simulink model "Kalman_builtin"  (R2024a)
settings: Solver=VariableStepAuto  StartTime=0.0  StopTime=10.0  RelTol=1e-3
undefined symbols (not defined in the file or in its folder): pInitialization
libraries: ctrlSharedLib x40, simulink x2
settings Model: Creator=DELL  LastModifiedBy=DELL

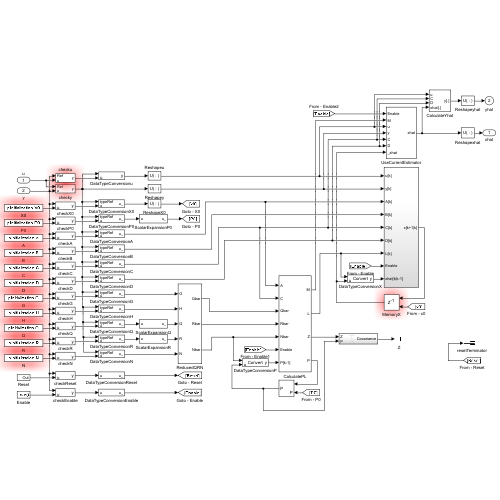
[thumbnail: Simulink's stored preview of the top-level diagram]
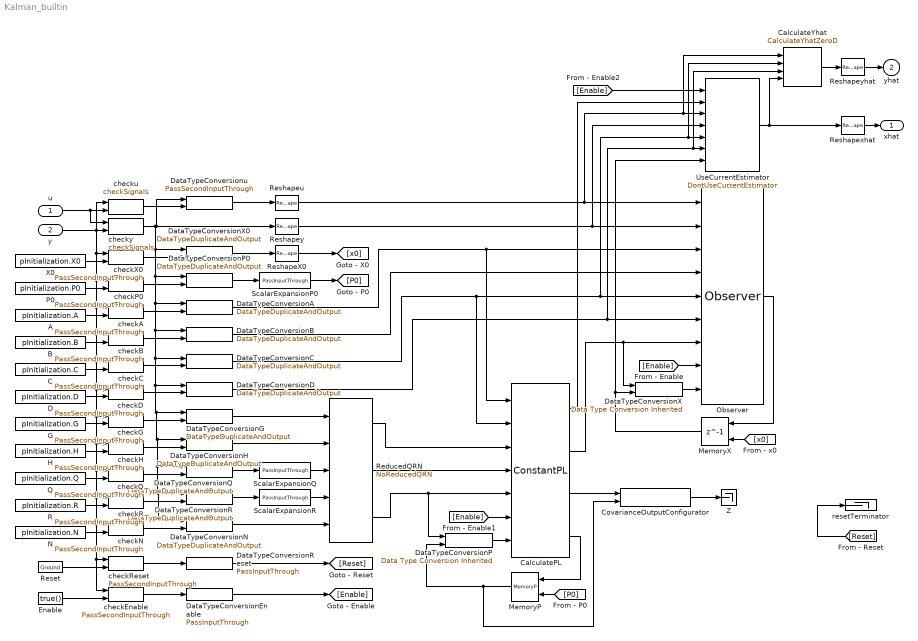
== system Kalman_builtin ==
  u : Inport
  y : Inport  Port=2
  A : Constant  Value=pInitialization.A  VectorParams1D=off  OutDataTypeStr=Inherit: Inherit via back propagation
  B : Constant  Value=pInitialization.B  VectorParams1D=off  OutDataTypeStr=Inherit: Inherit via back propagation
  C : Constant  Value=pInitialization.C  VectorParams1D=off  OutDataTypeStr=Inherit: Inherit via back propagation
  CalculatePL : ctrlSharedLib/KalmanFilterUtilities/ConstantPL  SystemSampleTime=-1  VariantActivationTime=update diagram  AllowFlexibleInterface=on  Latency=0  AutoFrameSizeCalculation=off
  CalculateYhat : ctrlSharedLib/KalmanFilterUtilities/CalculateYhatZeroD  SystemSampleTime=-1  VariantActivationTime=update diagram  AllowFlexibleInterface=on  Latency=0  AutoFrameSizeCalculation=off
  CovarianceOutputConfigurator : ctrlSharedLib/Kalman Filter/CovarianceOutputConfigurator  SystemSampleTime=-1  VariantActivationTime=update diagram  AllowFlexibleInterface=on  Latency=0  AutoFrameSizeCalculation=off
  D : Constant  Value=pInitialization.D  VectorParams1D=off  OutDataTypeStr=Inherit: Inherit via back propagation
  DataTypeConversionA : ctrlSharedLib/Utilities/DataTypeDuplicateAndOutput  SystemSampleTime=-1  VariantActivationTime=update diagram  AllowFlexibleInterface=on  Latency=0  AutoFrameSizeCalculation=off
  DataTypeConversionB : ctrlSharedLib/Utilities/DataTypeDuplicateAndOutput  SystemSampleTime=-1  VariantActivationTime=update diagram  AllowFlexibleInterface=on  Latency=0  AutoFrameSizeCalculation=off
  DataTypeConversionC : ctrlSharedLib/Utilities/DataTypeDuplicateAndOutput  SystemSampleTime=-1  VariantActivationTime=update diagram  AllowFlexibleInterface=on  Latency=0  AutoFrameSizeCalculation=off
  DataTypeConversionD : ctrlSharedLib/Utilities/DataTypeDuplicateAndOutput  SystemSampleTime=-1  VariantActivationTime=update diagram  AllowFlexibleInterface=on  Latency=0  AutoFrameSizeCalculation=off
  DataTypeConversionEnable : ctrlSharedLib/Utilities/PassInputThrough  SystemSampleTime=-1  VariantActivationTime=update diagram  AllowFlexibleInterface=on  Latency=0  AutoFrameSizeCalculation=off
  DataTypeConversionG : ctrlSharedLib/Utilities/DataTypeDuplicateAndOutput  SystemSampleTime=-1  VariantActivationTime=update diagram  AllowFlexibleInterface=on  Latency=0  AutoFrameSizeCalculation=off
  DataTypeConversionH : ctrlSharedLib/Utilities/DataTypeDuplicateAndOutput  SystemSampleTime=-1  VariantActivationTime=update diagram  AllowFlexibleInterface=on  Latency=0  AutoFrameSizeCalculation=off
  DataTypeConversionN : ctrlSharedLib/Utilities/DataTypeDuplicateAndOutput  SystemSampleTime=-1  VariantActivationTime=update diagram  AllowFlexibleInterface=on  Latency=0  AutoFrameSizeCalculation=off
  DataTypeConversionP : simulink/Signal Attributes/Data Type Conversion Inherited  ConvertRealWorld=Real World Value  DoSatur=off
  DataTypeConversionP0 : ctrlSharedLib/Utilities/DataTypeDuplicateAndOutput  SystemSampleTime=-1  VariantActivationTime=update diagram  AllowFlexibleInterface=on  Latency=0  AutoFrameSizeCalculation=off
  DataTypeConversionQ : ctrlSharedLib/Utilities/DataTypeDuplicateAndOutput  SystemSampleTime=-1  VariantActivationTime=update diagram  AllowFlexibleInterface=on  Latency=0  AutoFrameSizeCalculation=off
  DataTypeConversionR : ctrlSharedLib/Utilities/DataTypeDuplicateAndOutput  SystemSampleTime=-1  VariantActivationTime=update diagram  AllowFlexibleInterface=on  Latency=0  AutoFrameSizeCalculation=off
  DataTypeConversionReset : ctrlSharedLib/Utilities/PassInputThrough  SystemSampleTime=-1  VariantActivationTime=update diagram  AllowFlexibleInterface=on  Latency=0  AutoFrameSizeCalculation=off
  DataTypeConversionX : simulink/Signal Attributes/Data Type Conversion Inherited  ConvertRealWorld=Real World Value  DoSatur=off
  DataTypeConversionX0 : ctrlSharedLib/Utilities/DataTypeDuplicateAndOutput  SystemSampleTime=-1  VariantActivationTime=update diagram  AllowFlexibleInterface=on  Latency=0  AutoFrameSizeCalculation=off
  DataTypeConversionu : ctrlSharedLib/KalmanFilterUtilities/PassSecondInputThrough  SystemSampleTime=-1  VariantActivationTime=update diagram  AllowFlexibleInterface=on  Latency=0  AutoFrameSizeCalculation=off
  Enable : Constant  Value=true()  OutDataTypeStr=boolean
  G : Constant  Value=pInitialization.G  VectorParams1D=off  OutDataTypeStr=Inherit: Inherit via back propagation
  H : Constant  Value=pInitialization.H  VectorParams1D=off  OutDataTypeStr=Inherit: Inherit via back propagation
  MemoryP : ctrlSharedLib/KalmanFilterUtilities/MemoryP  SystemSampleTime=-1  VariantActivationTime=update diagram  AllowFlexibleInterface=on  Latency=0  AutoFrameSizeCalculation=off
  MemoryX : Delay  DelayLength=1  InitialConditionSource=Input port  SampleTime=pInitialization.Ts
      settings: InputPortMap=u0,p4
  N : Constant  Value=pInitialization.N  VectorParams1D=off  OutDataTypeStr=Inherit: Inherit via back propagation
  Observer : ctrlSharedLib/Kalman Filter/Observer  SystemSampleTime=-1  VariantActivationTime=update diagram  AllowFlexibleInterface=on  Latency=0  AutoFrameSizeCalculation=off
  P0 : Constant  Value=pInitialization.P0  OutDataTypeStr=Inherit: Inherit via back propagation
  Q : Constant  Value=pInitialization.Q  VectorParams1D=off  OutDataTypeStr=Inherit: Inherit via back propagation
  R : Constant  Value=pInitialization.R  VectorParams1D=off  OutDataTypeStr=Inherit: Inherit via back propagation
  ReducedQRN : ctrlSharedLib/KalmanFilterUtilities/NoReducedQRN  SystemSampleTime=-1  VariantActivationTime=update diagram  AllowFlexibleInterface=on  Latency=0  AutoFrameSizeCalculation=off
  Reset : ctrlSharedLib/Utilities/Ground  OutDataTypeStr=boolean  Dimensions=1
  ReshapeX0 : Reshape
  Reshapeu : Reshape
  Reshapexhat : Reshape
  Reshapey : Reshape
  Reshapeyhat : Reshape
  ScalarExpansionP0 : ctrlSharedLib/Utilities/PassInputThrough  SystemSampleTime=-1  VariantActivationTime=update diagram  AllowFlexibleInterface=on  Latency=0  AutoFrameSizeCalculation=off
  ScalarExpansionQ : ctrlSharedLib/Utilities/PassInputThrough  SystemSampleTime=-1  VariantActivationTime=update diagram  AllowFlexibleInterface=on  Latency=0  AutoFrameSizeCalculation=off
  ScalarExpansionR : ctrlSharedLib/Utilities/PassInputThrough  SystemSampleTime=-1  VariantActivationTime=update diagram  AllowFlexibleInterface=on  Latency=0  AutoFrameSizeCalculation=off
  UseCurrentEstimator : ctrlSharedLib/KalmanFilterUtilities/DontUseCurrentEstimator  SystemSampleTime=-1  VariantActivationTime=update diagram  AllowFlexibleInterface=on  Latency=0  AutoFrameSizeCalculation=off
  X0 : Constant  Value=pInitialization.X0  VectorParams1D=off  OutDataTypeStr=Inherit: Inherit via back propagation
  Z : Terminator
  checkA : ctrlSharedLib/KalmanFilterUtilities/PassSecondInputThrough  SystemSampleTime=-1  VariantActivationTime=update diagram  AllowFlexibleInterface=on  Latency=0  AutoFrameSizeCalculation=off
  checkB : ctrlSharedLib/KalmanFilterUtilities/PassSecondInputThrough  SystemSampleTime=-1  VariantActivationTime=update diagram  AllowFlexibleInterface=on  Latency=0  AutoFrameSizeCalculation=off
  checkC : ctrlSharedLib/KalmanFilterUtilities/PassSecondInputThrough  SystemSampleTime=-1  VariantActivationTime=update diagram  AllowFlexibleInterface=on  Latency=0  AutoFrameSizeCalculation=off
  checkD : ctrlSharedLib/KalmanFilterUtilities/PassSecondInputThrough  SystemSampleTime=-1  VariantActivationTime=update diagram  AllowFlexibleInterface=on  Latency=0  AutoFrameSizeCalculation=off
  checkEnable : ctrlSharedLib/KalmanFilterUtilities/PassSecondInputThrough  SystemSampleTime=-1  VariantActivationTime=update diagram  AllowFlexibleInterface=on  Latency=0  AutoFrameSizeCalculation=off
  checkG : ctrlSharedLib/KalmanFilterUtilities/PassSecondInputThrough  SystemSampleTime=-1  VariantActivationTime=update diagram  AllowFlexibleInterface=on  Latency=0  AutoFrameSizeCalculation=off
  checkH : ctrlSharedLib/KalmanFilterUtilities/PassSecondInputThrough  SystemSampleTime=-1  VariantActivationTime=update diagram  AllowFlexibleInterface=on  Latency=0  AutoFrameSizeCalculation=off
  checkN : ctrlSharedLib/KalmanFilterUtilities/PassSecondInputThrough  SystemSampleTime=-1  VariantActivationTime=update diagram  AllowFlexibleInterface=on  Latency=0  AutoFrameSizeCalculation=off
  checkP0 : ctrlSharedLib/KalmanFilterUtilities/PassSecondInputThrough  SystemSampleTime=-1  VariantActivationTime=update diagram  AllowFlexibleInterface=on  Latency=0  AutoFrameSizeCalculation=off
  checkQ : ctrlSharedLib/KalmanFilterUtilities/PassSecondInputThrough  SystemSampleTime=-1  VariantActivationTime=update diagram  AllowFlexibleInterface=on  Latency=0  AutoFrameSizeCalculation=off
  checkR : ctrlSharedLib/KalmanFilterUtilities/PassSecondInputThrough  SystemSampleTime=-1  VariantActivationTime=update diagram  AllowFlexibleInterface=on  Latency=0  AutoFrameSizeCalculation=off
  checkReset : ctrlSharedLib/KalmanFilterUtilities/PassSecondInputThrough  SystemSampleTime=-1  VariantActivationTime=update diagram  AllowFlexibleInterface=on  Latency=0  AutoFrameSizeCalculation=off
  checkX0 : ctrlSharedLib/KalmanFilterUtilities/PassSecondInputThrough  SystemSampleTime=-1  VariantActivationTime=update diagram  AllowFlexibleInterface=on  Latency=0  AutoFrameSizeCalculation=off
  checku : ctrlSharedLib/KalmanFilterUtilities/checkSignals  Ts=pInitialization.Ts  Ns=pInitialization.Ns  Nu=pInitialization.Nu  Nw=pInitialization.Nw  Ny=pInitialization.Ny
  checky : ctrlSharedLib/KalmanFilterUtilities/checkSignals  Ts=pInitialization.Ts  Ns=pInitialization.Ns  Nu=pInitialization.Nu  Nw=pInitialization.Nw  Ny=pInitialization.Ny
  resetTerminator : Terminator
  xhat : Outport  VectorParamsAs1DForOutWhenUnconnected=off
  yhat : Outport  Port=2
  wires:
  checkG/1 -> DataTypeConversionG/2
  C/1 -> checkC/2
  ReducedQRN/3 -> CalculatePL/5, DataTypeConversionP/1
  CalculatePL/1 -> UseCurrentEstimator/2
  D/1 -> checkD/2
  checkR/1 -> DataTypeConversionR/2
  checkC/1 -> DataTypeConversionC/2
  G/1 -> checkG/2
  y/1 -> checky/2, checku/1, checkX0/1, checkP0/1, checkA/1, checkB/1, checkC/1, checkD/1, checkG/1, checkH/1, checkQ/1, checkR/1, checkN/1, checkReset/1, checkEnable/1
  DataTypeConversionN/1 -> ReducedQRN/5
  Q/1 -> checkQ/2
  H/1 -> checkH/2
  DataTypeConversionX0/1 -> ReshapeX0/1
  DataTypeConversionD/1 -> Observer/6, UseCurrentEstimator/6, CalculateYhat/3
  [P0] -> MemoryP/2
  DataTypeConversionG/1 -> ReducedQRN/1
  checkN/1 -> DataTypeConversionN/2
  Observer/1 -> MemoryX/1
  DataTypeConversionA/1 -> Observer/3, CalculatePL/1
  DataTypeConversionReset/1 -> [Reset]
  [Enable] -> CalculatePL/6
  checkQ/1 -> DataTypeConversionQ/2
  DataTypeConversionC/1 -> Observer/5, UseCurrentEstimator/5, CalculateYhat/2, CalculatePL/2
  DataTypeConversionQ/1 -> ScalarExpansionQ/1
  checkD/1 -> DataTypeConversionD/2
  DataTypeConversionEnable/1 -> [Enable]
  N/1 -> checkN/2
  Reshapexhat/1 -> xhat/1
  Enable/1 -> checkEnable/2
  DataTypeConversionP0/1 -> ScalarExpansionP0/1
  DataTypeConversionR/1 -> ScalarExpansionR/1
  Reset/1 -> checkReset/2
  DataTypeConversionP/1 -> CalculatePL/7
  u/1 -> checku/2, checky/1
  checkEnable/1 -> DataTypeConversionEnable/1
  checkH/1 -> DataTypeConversionH/2
  [Enable] -> Observer/8
  X0/1 -> checkX0/2
  A/1 -> checkA/2
  checkA/1 -> DataTypeConversionA/2
  Reshapeu/1 -> Observer/1, UseCurrentEstimator/3, CalculateYhat/1
  checkB/1 -> DataTypeConversionB/2
  DataTypeConversionX/1 -> Observer/9
  DataTypeConversionB/1 -> Observer/4
  CalculatePL/4 -> MemoryP/1
  Reshapey/1 -> Observer/2, UseCurrentEstimator/4
  MemoryP/1 -> DataTypeConversionP/2, CovarianceOutputConfigurator/2
  checky/1 -> DataTypeConversionX0/1, DataTypeConversionP0/1, DataTypeConversionC/1, DataTypeConversionD/1, DataTypeConversionG/1, DataTypeConversionH/1, DataTypeConversionQ/1, DataTypeConversionR/1, DataTypeConversionN/1, DataTypeConversionB/1, DataTypeConversionA/1, Reshapey/1, DataTypeConversionu/1
  ReshapeX0/1 -> [x0]
  checkP0/1 -> DataTypeConversionP0/2
  CalculateYhat/1 -> Reshapeyhat/1
  ReducedQRN/2 -> CalculatePL/4
  [Enable] -> UseCurrentEstimator/1
  B/1 -> checkB/2
  checkReset/1 -> DataTypeConversionReset/1
  ScalarExpansionR/1 -> ReducedQRN/4
  ScalarExpansionP0/1 -> [P0]
  ScalarExpansionQ/1 -> ReducedQRN/3
  MemoryX/1 -> DataTypeConversionX/2, UseCurrentEstimator/7
  DataTypeConversionH/1 -> ReducedQRN/2
  R/1 -> checkR/2
  CovarianceOutputConfigurator/1 -> Z/1
  P0/1 -> checkP0/2
  Reshapeyhat/1 -> yhat/1
  [Reset] -> resetTerminator/1
  checku/1 -> DataTypeConversionu/2
  CalculatePL/3 -> CovarianceOutputConfigurator/1
  UseCurrentEstimator/1 -> Reshapexhat/1, CalculateYhat/4
  ReducedQRN/1 -> CalculatePL/3
  CalculatePL/2 -> Observer/7, DataTypeConversionX/1
  DataTypeConversionu/1 -> Reshapeu/1
  checkX0/1 -> DataTypeConversionX0/2
  [x0] -> MemoryX/2
